simulink library "RoomWithRadiatorAndUFP"  (R2025a)
settings: Solver=VariableStepAuto  StartTime=0.0  StopTime=10.0  RelTol=1e-3
libraries: fl_lib x10, RoomUnderFloorPiping_lib x1, RoomVolume_lib x1, RoomRadiator_lib x1
settings Model: Creator=vikrants  LastModifiedBy=vikrants

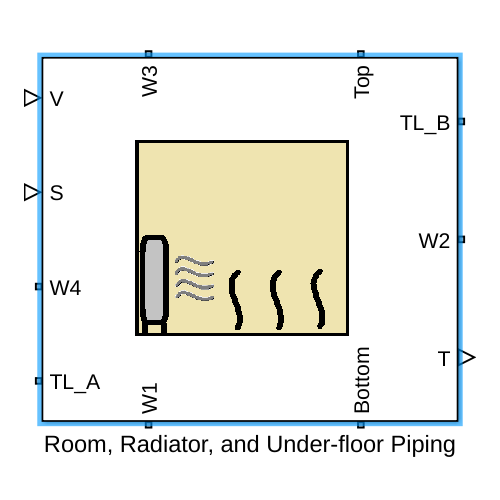
[thumbnail: Simulink's stored preview of the top-level diagram]
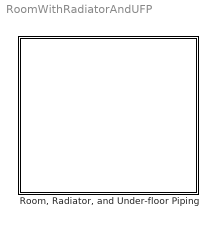
== system RoomWithRadiatorAndUFP ==
  "Room, Radiator, and Under-floor Piping" : Subsystem  mask{pipeRoughnessR=1e-6, pipeLenR=10, pipeCrossSectionalAreaR=1.75e-4, pipeHydrDiaR=1.5e-2, pipeRoughnessUFP=1e-6, pipeLenUFP=50, pipeCrossSectionalAreaUFP=1.75e-4, pipeHydrDiaUFP=1.5e-2, thermalResFloor=100, roomWid=3, roomHgt=2.5, roomLen=5, htc=10, iniT=300, indxS=1, indxV=1}
      mask prompts: pipeRoughnessR "Pipe roughness (m)"; pipeLenR "Pipe length (m)"; pipeCrossSectionalAreaR "Pipe cross-sectional area (m^2)"; pipeHydrDiaR "Pipe hydraulic diameter (m)"; pipeRoughnessUFP "Pipe roughness (m)"; pipeLenUFP "Pipe length (m)"; pipeCrossSectionalAreaUFP "Pipe cross-sectional area (m^2)"; pipeHydrDiaUFP "Pipe hydraulic diameter (m)"; thermalResFloor "Thermal resistance to floor (K/W)"; roomWid "Room Width (m)"; roomHgt "Room Height (m)"; roomLen "Room Length (m)"; htc "Heat Transfer Coefficient (W/K*m^2)"; iniT "Initial Temperature (K)"; indxS "Heat source vector index"; indxV "Valve operation vector index"
      settings: PortSchema="{\"entries\":[{\"content\":{\"sides\":[{\"content\":{\"connectorIds\":[\"LConn1\",\"LConn2\",\"LConn3\",\"LConn4\"]},\"type\":\"ConnectorPlacement.EquallySpacedRectSide\",\"uuid\":\"8440f6ae-3089-4f14-af97-f7a7d9c670fb\"},{\"content\":{\"connectorIds\":[\"RConn1\",\"RConn2\",\"RConn3\"],\"side\":\"RIGHT\"},\"type\":\"ConnectorPlacement.EquallySpacedRectSide\",\"uuid\":\"df84a625-bd6d-46a4-b71c-d411d28f8df6\"},{\"content\":{\"connectorIds\":[\"LConn5\",\"LConn6\"],\"side\":\"TOP\"},\"type\":\"ConnectorPlacement.EquallySpacedRectSide\",\"uuid\":\"90f16a0a-d00c-4f13-8e79-f2f23ea8b565\"},{\"content\":{\"connectorIds\":[\"RConn4\",\"RConn5\"],\"side\":\"BOTTOM\"},\"type\":\"ConnectorPlacement.EquallySpacedRectSide\",\"uuid\":\"4eb9d9d9-e9b4-43a3-a1e1-726815f3b9ff\"}]},\"type\":\"ConnectorPlacement.EquallySpacedConnector\",\"uuid\":\"51dc529f-94b8-407e-b287-301b2c0c8383\"}],\"packageUris\":[\"http://schema.mathworks.com/mf0/Connector/R2020b\"],\"version\":\"1.0\"}"
      mask Help: web("DocumentationCompositeRoomRadiatorUFP.html")
      mask DialogControl DescGroupVar Prompt: Description
      mask DialogControl DescTextVar Prompt: Room model with radiator and under-floor piping for thermal comfort.
      mask DialogControl ParameterGroupRadiator Prompt: Radiator
      mask DialogControl ParameterGroupUFP Prompt: Under Floor Piping
      mask DialogControl ParameterGroupRoom Prompt: Room Dimensions
      mask DialogControl ParameterGroupHT Prompt: Heat Transfer
      mask Display: image("roomWithRadiatorAndUFP.png");

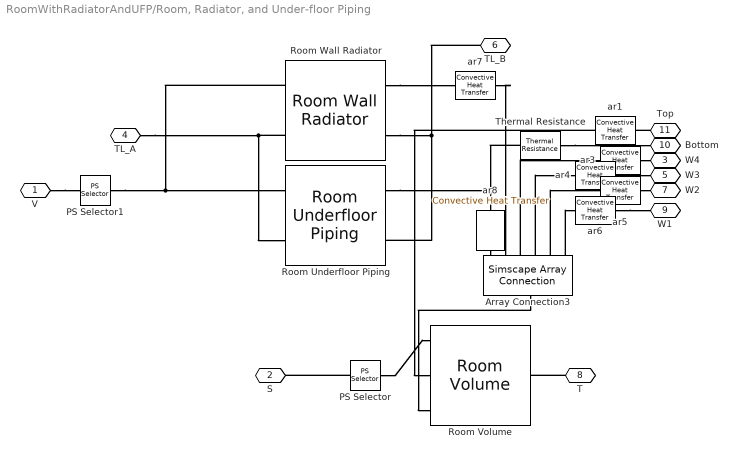
== system RoomWithRadiatorAndUFP/Room, Radiator, and Under-floor Piping ==
  Array Connection3 : SimscapeArrayConnection  Domain=foundation.thermal.thermal  NumScalarElements=6
  PS Selector : fl_lib/Physical Signals/Nonlinear Operators/PS Selector  ix=indxS
      settings: InternalSimscapePortConfiguration="{\"Bottom\":[],\"Left\":[{\"id\":\"I\",\"label\":\"\",\"type\":\"input\"}],\"Right\":[{\"id\":\"O\",\"label\":\"\",\"type\":\"output\"}],\"Top\":[]}"
  PS Selector1 : fl_lib/Physical Signals/Nonlinear Operators/PS Selector  ix=indxV
      settings: InternalSimscapePortConfiguration="{\"Bottom\":[],\"Left\":[{\"id\":\"I\",\"label\":\"\",\"type\":\"input\"}],\"Right\":[{\"id\":\"O\",\"label\":\"\",\"type\":\"output\"}],\"Top\":[]}"
  Room Underfloor Piping : RoomUnderFloorPiping_lib/Room Underfloor Piping  pipeHydrDia=pipeHydrDiaUFP m  pipeLength=pipeLenUFP m  pipeArea=pipeCrossSectionalAreaUFP m^2  pipeRoughness=pipeRoughnessUFP m  htc=htc W/(K*m^2)  iniTemperature=iniT K
      settings: InternalSimscapePortConfiguration="{\"Bottom\":[],\"Left\":[{\"id\":\"TL_V\",\"label\":\"V\",\"type\":\"input\"},{\"id\":\"TL_A\",\"label\":\"A\",\"type\":\"foundation.thermal_liquid.thermal_liquid\"}],\"Right\":[{\"id\":\"M\",\"label\":\"R\",\"type\":\"foundation.thermal.thermal\"},{\"id\":\"TL_B\",\"label\":\"B\",\"type\":\"foundation.thermal_liquid.thermal_liquid\"}],\"Top\":[]}"
  Room Volume : RoomVolume_lib/Room Volume  N1=1  N2=6  iniT=iniT K  length=roomLen m  width=roomWid m  height=roomHgt m
      settings: InternalSimscapePortConfiguration="{\"Bottom\":[],\"Left\":[{\"id\":\"S\",\"label\":\"S\",\"type\":\"input\"}],\"Right\":[{\"id\":\"T\",\"label\":\"T\",\"type\":\"output\"}],\"Top\":[{\"id\":\"M1\",\"label\":\"M1\",\"type\":\"foundation.thermal.thermal\"},{\"id\":\"M2\",\"label\":\"M2\",\"type\":\"foundation.thermal.thermal\"}]}"
  Room Wall Radiator : RoomRadiator_lib/Room Wall Radiator  pipeHydrDia=pipeHydrDiaR m  pipeLength=pipeLenR m  pipeArea=pipeCrossSectionalAreaR m^2  pipeRoughness=pipeRoughnessR m  htc=htc W/(K*m^2)  iniTemperature=iniT K
      settings: InternalSimscapePortConfiguration="{\"Bottom\":[],\"Left\":[{\"id\":\"TL_V\",\"label\":\"V\",\"type\":\"input\"},{\"id\":\"TL_A\",\"label\":\"A\",\"type\":\"foundation.thermal_liquid.thermal_liquid\"}],\"Right\":[{\"id\":\"M\",\"label\":\"R\",\"type\":\"foundation.thermal.thermal\"},{\"id\":\"TL_B\",\"label\":\"B\",\"type\":\"foundation.thermal_liquid.thermal_liquid\"}],\"Top\":[]}"
  Thermal Resistance : fl_lib/Thermal/Thermal Elements/Thermal Resistance  resistance=thermalResFloor K/W  T_specify=off  T_priority=None  T=0 K  T_nominal_specify=off  T_nominal_value=1  T_nominal_unit=K  Q_specify=off  Q_priority=None  Q=0 W  Q_nominal_specify=off  Q_nominal_value=1  Q_nominal_unit=W
  ar1 : fl_lib/Thermal/Thermal Elements/Convective Heat Transfer  thermal_type=foundation.enum.constant_variable.constant  area=roomLen*roomWid m^2  heat_tr_coeff=htc W/(K*m^2)  min_heat_tr_coeff=1e-3 W/(K*m^2)  T_specify=off  T_priority=None  T=0 K  T_nominal_specify=off  T_nominal_value=1  T_nominal_unit=K  Q_specify=off  Q_priority=None  Q=0 W  Q_nominal_specify=off  Q_nominal_value=1  Q_nominal_unit=W
  ar3 : fl_lib/Thermal/Thermal Elements/Convective Heat Transfer  thermal_type=foundation.enum.constant_variable.constant  area=roomHgt*roomWid m^2  heat_tr_coeff=htc W/(K*m^2)  min_heat_tr_coeff=1e-3 W/(K*m^2)  T_specify=off  T_priority=None  T=0 K  T_nominal_specify=off  T_nominal_value=1  T_nominal_unit=K  Q_specify=off  Q_priority=None  Q=0 W  Q_nominal_specify=off  Q_nominal_value=1  Q_nominal_unit=W
  ar4 : fl_lib/Thermal/Thermal Elements/Convective Heat Transfer  thermal_type=foundation.enum.constant_variable.constant  area=roomLen*roomHgt m^2  heat_tr_coeff=htc W/(K*m^2)  min_heat_tr_coeff=1e-3 W/(K*m^2)  T_specify=off  T_priority=None  T=0 K  T_nominal_specify=off  T_nominal_value=1  T_nominal_unit=K  Q_specify=off  Q_priority=None  Q=0 W  Q_nominal_specify=off  Q_nominal_value=1  Q_nominal_unit=W
  ar5 : fl_lib/Thermal/Thermal Elements/Convective Heat Transfer  thermal_type=foundation.enum.constant_variable.constant  area=roomHgt*roomWid m^2  heat_tr_coeff=htc W/(K*m^2)  min_heat_tr_coeff=1e-3 W/(K*m^2)  T_specify=off  T_priority=None  T=0 K  T_nominal_specify=off  T_nominal_value=1  T_nominal_unit=K  Q_specify=off  Q_priority=None  Q=0 W  Q_nominal_specify=off  Q_nominal_value=1  Q_nominal_unit=W
  ar6 : fl_lib/Thermal/Thermal Elements/Convective Heat Transfer  thermal_type=foundation.enum.constant_variable.constant  area=roomLen*roomHgt m^2  heat_tr_coeff=htc W/(K*m^2)  min_heat_tr_coeff=1e-3 W/(K*m^2)  T_specify=off  T_priority=None  T=0 K  T_nominal_specify=off  T_nominal_value=1  T_nominal_unit=K  Q_specify=off  Q_priority=None  Q=0 W  Q_nominal_specify=off  Q_nominal_value=1  Q_nominal_unit=W
  ar7 : fl_lib/Thermal/Thermal Elements/Convective Heat Transfer  thermal_type=foundation.enum.constant_variable.constant  area=pipeLenR*pipeHydrDiaR m^2  heat_tr_coeff=htc W/(K*m^2)  min_heat_tr_coeff=1e-3 W/(K*m^2)  T_specify=off  T_priority=None  T=0 K  T_nominal_specify=off  T_nominal_value=1  T_nominal_unit=K  Q_specify=off  Q_priority=None  Q=0 W  Q_nominal_specify=off  Q_nominal_value=1  Q_nominal_unit=W
  ar8 : fl_lib/Thermal/Thermal Elements/Convective Heat Transfer  thermal_type=foundation.enum.constant_variable.constant  area=pipeLenUFP*pipeHydrDiaUFP/2 m^2  heat_tr_coeff=htc W/(K*m^2)  min_heat_tr_coeff=1e-3 W/(K*m^2)  T_specify=off  T_priority=None  T=0 K  T_nominal_specify=off  T_nominal_value=1  T_nominal_unit=K  Q_specify=off  Q_priority=None  Q=0 W  Q_nominal_specify=off  Q_nominal_value=1  Q_nominal_unit=W
  V : PMIOPort  Side=Left
  S : PMIOPort  Port=2  Side=Left
  W4 : PMIOPort  Port=3  Side=Left
  TL_A : PMIOPort  Port=4  Side=Left
  W3 : PMIOPort  Port=5  Side=Left
  TL_B : PMIOPort  Port=6  Side=Right
  W2 : PMIOPort  Port=7  Side=Right
  T : PMIOPort  Port=8  Side=Right
  W1 : PMIOPort  Port=9  Side=Right
  Bottom : PMIOPort  Port=10  Side=Right
  Top : PMIOPort  Port=11  Side=Left
  connections:
  Array Connection3/RConn1 -- Room Volume/LConn3
  TL_B/RConn1 -- Room Wall Radiator/RConn2 -- Room Underfloor Piping/RConn2
  T/RConn1 -- Room Volume/RConn1
  TL_A/RConn1 -- Room Wall Radiator/LConn2 -- Room Underfloor Piping/LConn2
  ar6/RConn1 -- W1/RConn1
  ar5/RConn1 -- W2/RConn1
  ar4/RConn1 -- W3/RConn1
  ar3/RConn1 -- W4/RConn1
  Room Underfloor Piping/RConn1 -- Thermal Resistance/LConn1 -- ar8/LConn1
  ar7/RConn1 -- Array Connection3/LConn2
  ar1/LConn1 -- Room Volume/LConn2
  Top/RConn1 -- ar1/RConn1
  Thermal Resistance/RConn1 -- Bottom/RConn1
  Array Connection3/LConn3 -- ar3/LConn1
  Array Connection3/LConn4 -- ar4/LConn1
  Array Connection3/LConn5 -- ar5/LConn1
  Array Connection3/LConn6 -- ar6/LConn1
  Room Wall Radiator/RConn1 -- ar7/LConn1
  ar8/RConn1 -- Array Connection3/LConn1
  V/RConn1 -- PS Selector1/LConn1
  PS Selector1/RConn1 -- Room Wall Radiator/LConn1 -- Room Underfloor Piping/LConn1
  PS Selector/RConn1 -- Room Volume/LConn1
  PS Selector/LConn1 -- S/RConn1
